simulink model "CruiseControlSimClose"  (R2024a)
settings: Solver=ode45  StartTime=0.0  StopTime=50  MaxStep=1e-3  RelTol=1e-3
values from neighbouring files (symbols this model uses):
  b0 = -336.4    [CruiseControlPlots.m]
  b1 = 23.2    [CruiseControlPlots.m]
  Fgrav = 1400    [CruiseControlPlots.m]
  Froll = 228    [CruiseControlPlots.m]
  k = 40    [CruiseControlPlots.m]
  ki = 4.69    [CruiseControlPlots.m]    (also in hw3problem1.m = 125)
  kp = 30.7    [CruiseControlPlots.m]    (also in hw3problem1.m = 73)
  m = 2085    [CruiseControlPlots.m]
  ubar = (b1 * 29 + (Froll + b0)) / k    (= 14.11)    [CruiseControlPlots.m]
  v0 = 29    [CruiseControlPlots.m]
  v_des = 29    [CruiseControlPlots.m]
settings Model: Creator=xinchen  LastModifiedBy=xinchen

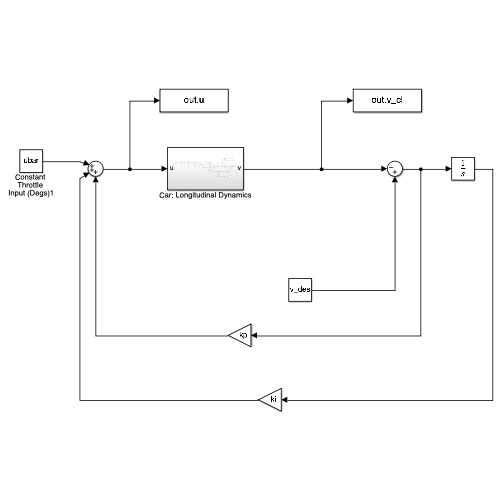
[thumbnail: Simulink's stored preview of the top-level diagram]
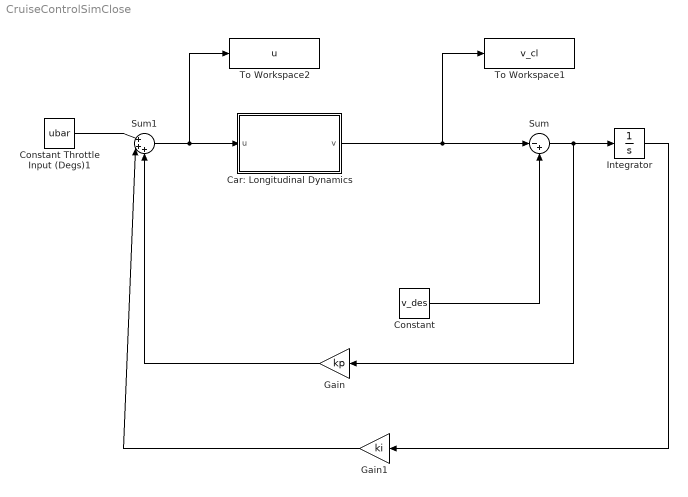
== system CruiseControlSimClose ==
  Car: Longitudinal Dynamics : Subsystem
  Constant : Constant  Value=v_des
  Constant Throttle Input (Degs)1 : Constant  Value=ubar
  Gain : Gain  Gain=kp
  Gain1 : Gain  Gain=ki
  Integrator : Integrator
  Sum : Sum  Inputs=|-+
  Sum1 : Sum  Inputs=|+++
  To Workspace1 : ToWorkspace  VariableName=v_cl  SampleTime=-1
  To Workspace2 : ToWorkspace  VariableName=u  SampleTime=-1
  wires:
  Sum/1 -> Integrator/1, Gain/1
  Car: Longitudinal Dynamics/1(v) -> Sum/1, To Workspace1/1
  Constant Throttle Input (Degs)1/1 -> Sum1/1
  Integrator/1 -> Gain1/1
  Gain1/1 -> Sum1/2
  Gain/1 -> Sum1/3
  Constant/1 -> Sum/2
  Sum1/1 -> To Workspace2/1, Car: Longitudinal Dynamics/1(u)

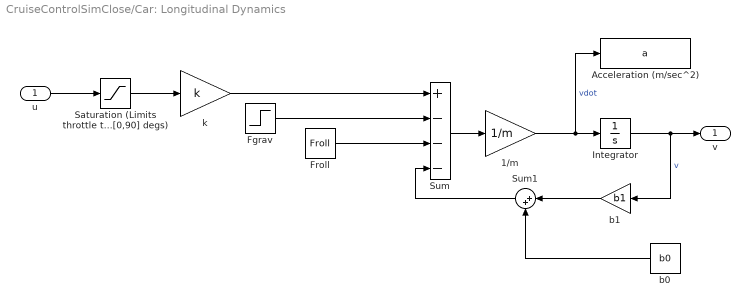
== system CruiseControlSimClose/Car: Longitudinal Dynamics ==
  u : Inport
  1/m : Gain  Gain=1/m
  Acceleration (m/sec^2) : ToWorkspace  VariableName=a  SampleTime=-1
  Fgrav : Step  Time=10  After=Fgrav  SampleTime=0
  Froll : Constant  Value=Froll
  Integrator : Integrator  InitialCondition=v0
  Saturation (Limits throttle to [0,90] degs) : Saturate  UpperLimit=90  LowerLimit=0
  Sum : Sum  Inputs=+---
  Sum1 : Sum  Inputs=|++
  b0 : Constant  Value=b0
  b1 : Gain  Gain=b1
  k : Gain  Gain=k
  v : Outport
  wires:
  Sum1/1 -> Sum/4
  Froll/1 -> Sum/3
  Fgrav/1 -> Sum/2
  k/1 -> Sum/1
  b0/1 -> Sum1/2
  b1/1 -> Sum1/1
  u/1 -> Saturation (Limits throttle to [0,90] degs)/1
  Sum/1 -> 1/m/1
  Integrator/1 -> v/1, b1/1  "v"
  1/m/1 -> Acceleration (m/sec^2)/1, Integrator/1  "vdot"
  Saturation (Limits throttle to [0,90] degs)/1 -> k/1
